simulink model "test_hh_neuron"  (R2018a)
settings: Solver=VariableStepAuto  StartTime=0.0  StopTime=100  MaxStep=1e-2  RelTol=1e-3
libraries: fl_lib x8, nesl_utility x2
settings Model: Creator=bici  LastModifiedBy=bici
settings DataIOCC: SaveState=on  InspectSignalLogs=on

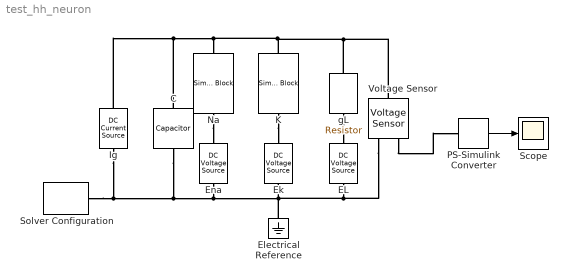
== system test_hh_neuron ==
  C : fl_lib/Electrical/Electrical Elements/Capacitor  c=1 uF  r=0 Ohm  g=0 1/Ohm  i_specify=off  i_priority=None  i=0 A  i_nominal_specify=off  i_nominal_unit=A  i_nominal_value=1  v_specify=off  v_priority=None  v=-10 mV  v_nominal_specify=off  v_nominal_unit=V  v_nominal_value=1  vc_specify=on  vc_priority=High  vc=-10 mV  vc_nominal_specify=off  vc_nominal_unit=V  vc_nominal_value=1
  EL : fl_lib/Electrical/Electrical Sources/DC Voltage Source  v0=10.6 mV
  Ek : fl_lib/Electrical/Electrical Sources/DC Voltage Source  v0=-12 mV
  Electrical Reference : fl_lib/Electrical/Electrical Elements/Electrical Reference
  Ena : fl_lib/Electrical/Electrical Sources/DC Voltage Source  v0=115 mV
  Ig : fl_lib/Electrical/Electrical Sources/DC Current Source  i0=5 uA
      settings: SourceProductName=Simscape  SourceProductBaseCode=SS
  K : SimscapeComponentBlock  SourceFile=memristor_hh_k_v2  ComponentPath=memristor_hh_k_v2  ComponentVariants=memristor_hh_k_v2  ComponentVariantNames=memristor_hh_k_v2  ClassName=memristor_hh_k_v2  SchemaVersion=1  g=36 mS  E=-12 mV  i_specify=off  i_priority=None  i=0 A  i_nominal_specify=off  i_nominal_unit=A  i_nominal_value=1  v_specify=off  v_priority=None  v=0 V  v_nominal_specify=off  v_nominal_unit=V  v_nominal_value=1
      settings: CopyFcn=simscape.engine.sli.internal.componentblockcallback(gcbh,'COPY')  PreCopyFcn=simscape.engine.sli.internal.componentblockcallback(gcbh,'PRECOPY')  PreDeleteFcn=simscape.engine.sli.internal.componentblockcallback(gcbh,'PREDELETE')
      mask Type: Hodzkin-Hakslijev kalijumov memristor
  Na : SimscapeComponentBlock  SourceFile=memristor_hh_na_v2  ComponentPath=memristor_hh_na_v2  ComponentVariants=memristor_hh_na_v2  ComponentVariantNames=memristor_hh_na_v2  ClassName=memristor_hh_na_v2  SchemaVersion=1  g=120 mS  E=115 mV  i_specify=off  i_priority=None  i=0 A  i_nominal_specify=off  i_nominal_unit=A  i_nominal_value=1  v_specify=off  v_priority=None  v=0 V  v_nominal_specify=off  v_nominal_unit=V  v_nominal_value=1
      settings: CopyFcn=simscape.engine.sli.internal.componentblockcallback(gcbh,'COPY')  PreCopyFcn=simscape.engine.sli.internal.componentblockcallback(gcbh,'PRECOPY')  PreDeleteFcn=simscape.engine.sli.internal.componentblockcallback(gcbh,'PREDELETE')
      mask Type: Hodzkin-Hakslijev natrijumov memristor
  PS-Simulink Converter : nesl_utility/PS-Simulink Converter  PhysicalDomain=network_engine_domain  SubClassName=ps_output  LeftPortType=input  RightPortType=output  PseudoPeriodic=off  Frequencies=[]  Unit=1  AffineConversion=off
  Scope : Scope
  Solver Configuration : nesl_utility/Solver Configuration  PhysicalDomain=network_engine_domain  SubClassName=solver  LeftPortType=input  RightPortType=generic  Tones=[]  Harmonics=[]  SimulateNoise=off  Profile=off  UseLocalSampling=off  EnableSwitchedLinearOptims=on  FrequencyDomain=off  UseCCode=off  RelTol=0.001  AbsTol=1e-06  MinStep=1e-09  ToWorkspace=off  RevertToSquareIcSolve=off  NumHomotopyIterations=100  PhasorMode=off  PhasorModeNumHarmonics=1  DoDC=off  ResidualTolerance=1e-09  UseLocalSolver=off  LocalSolverChoice=NE_BACKWARD_EULER_ADVANCER  LocalSolverSampleTime=0.001  DoFixedCost=off  MaxNonlinIter=3  MaxModeIter=2  LinearAlgebra=Sparse  EquationFormulation=NE_TIME_EF  DelaysMemoryBudget=1024  AutomaticFiltering=on  FilteringTimeConstant=0.001
  Voltage Sensor : fl_lib/Electrical/Electrical Sensors/Voltage Sensor
  gL : fl_lib/Electrical/Electrical Elements/Resistor  R=1/0.0003 Ohm  i_specify=off  i_priority=None  i=0 A  i_nominal_specify=off  i_nominal_unit=A  i_nominal_value=1  v_specify=off  v_priority=None  v=40 mV  v_nominal_specify=off  v_nominal_unit=V  v_nominal_value=1
  wires:
  PS-Simulink Converter/1 -> Scope/1
  connections:
  Electrical Reference/LConn1 -- Voltage Sensor/RConn2 -- EL/RConn1 -- Ig/RConn1 -- Solver Configuration/RConn1 -- C/RConn1 -- Ena/RConn1 -- Ek/RConn1
  gL/RConn1 -- EL/LConn1
  Na/RConn1 -- Ena/LConn1
  K/RConn1 -- Ek/LConn1
  C/LConn1 -- Ig/LConn1 -- Voltage Sensor/LConn1 -- gL/LConn1 -- K/LConn1 -- Na/LConn1
  Voltage Sensor/RConn1 -- PS-Simulink Converter/LConn1
